simulink model "OpenLoop_TF_Asynch_Driver"  (R2021b)
settings: Solver=ode23s  StartTime=0.0  StopTime=10.0  MaxStep=10e-4  RelTol=1e-3  EnableMultiTasking=on
libraries: spsUniversalBridgeLib x2, spsVoltageMeasurementLib x2, spsAsynchronousMachineSIUnitsLib x1, spsCurrentMeasurementLib x1, spsPWMGenerator2LevelLib x1, spsRMSLib x1, simulink x1, spsSeriesRLCBranchLib x1, spsThreePhaseProgrammableVoltageSourceLib x1, spspowerguiLib x1
settings Model: Creator=Mostafa  LastModifiedBy=Unicorn
settings SolverCC: AlgebraicLoopSolver=TrustRegion
settings DataIOCC: ReturnWorkspaceOutputs=off
settings OptimizationCC: LifeSpan=inf
settings DebuggingCC: SFUnexpectedBacktrackingDiag=warning  SFNoUnconditionalDefaultTransitionDiag=warning  SFMachineParentedDataDiag=warning  ArithmeticOperatorsInVariantConditions=warning
settings SFSimCC: SimUseLocalCustomCode=off  CustomCodeUndefinedFunction=UseInterfaceOnly
settings RTWCC: RTWUseLocalCustomCode=off
settings CodeAppCC: StateflowObjectComments=on
settings GRTTargetCC: TargetLangStandard=C89/C90 (ANSI)
settings ConfigComp: CovMetricSettings=dw  CovSaveCumulativeToWorkspaceVar=on  CovSaveSingleToWorkspaceVar=on  CovExternalEMLEnable=off
settings SimscapeCC: SimscapeNormalizeSystem=off

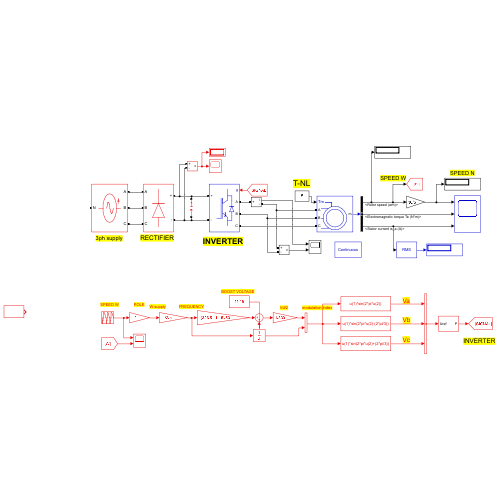
[thumbnail: Simulink's stored preview of the top-level diagram]
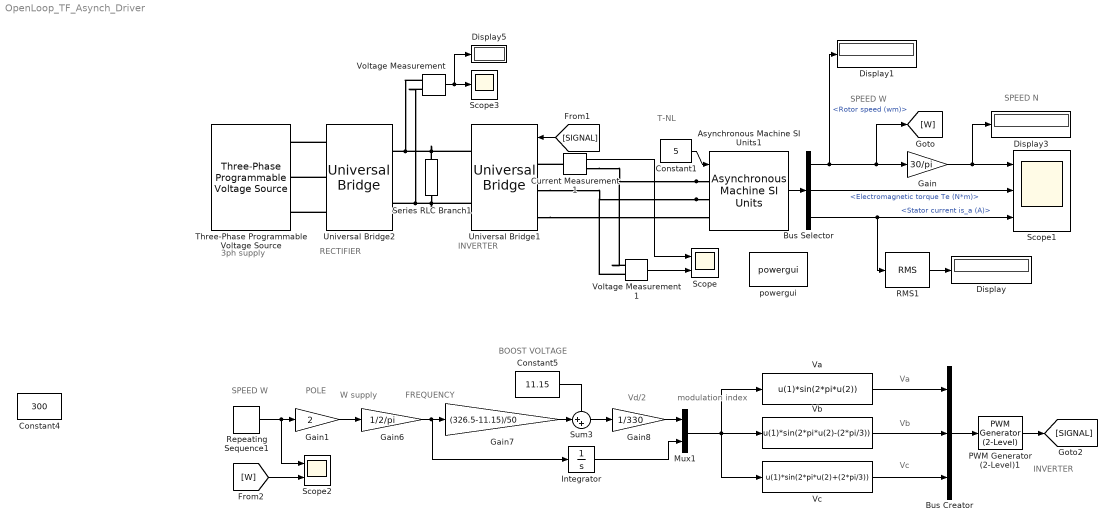
== system OpenLoop_TF_Asynch_Driver ==
  note: INVERTER
  note: Va
  note: RECTIFIER
  note: 3ph supply
  note: INVERTER
  note: T-NL
  note: SPEED W
  note: SPEED N
  note: POLE
  note: W supply
  note: BOOST VOLTAGE
  note: FREQUENCY
  note: SPEED W
  note: Vd/2
  note: modulation index
  note: Vb
  note: Vc
  Asynchronous Machine SI Units1 : spsAsynchronousMachineSIUnitsLib/Asynchronous Machine SI Units  RotorType=Squirrel-cage  PresetModel="15:  5.4 HP (4KW)   400 V  50Hz 1430 RPM"  MechanicalLoad=Torque Tm  ShowDetailedParameters=on  ReferenceFrame=Rotor  Units=SI  MeasurementBus=off  NominalParameters=[4000 400 50]  VoltageRatio=1  Stator=[1.405 0.005839]  Rotor=[1.395 0.005839]  Cage1=[0.4155 0.002066]  Cage2=[0.4168 0.0003495]  Lm=0.1722  Mechanical=[0.0131 0.002985 2]  PolePairs=2  InitialConditions=[1 0 0 0 0 0 0 0]  SimulateSaturation=off  Saturation=[14.03593122, 27.81365428, 53.79336849, 72.68890987, 97.98006896, 148.6815601, 215.7428561, 302.9841135, 428.7778367 ; 230, 322, 414, 460, 506, 552, 598, 644, 690]  LoadFlowParameters=1492000  TsPowergui=0  TsBlock=-1  IterativeModel=Trapezoidal non iterative  IterativeDiscreteModel=Trapezoidal non iterative  Pmec=1.492e+006
  Bus Creator : BusCreator  Inputs=3
  Bus Selector : BusSelector  OutputSignals=Mechanical.Rotor speed (wm),Mechanical.Electromagnetic torque Te (N*m),Stator measurements.Stator current is_a (A)
  Constant1 : Constant  Value=5
  Constant4 : Constant  Value=300
  Constant5 : Constant  Value=11.15
  Current Measurement1 : spsCurrentMeasurementLib/Current Measurement  PhasorSimulation=off  OutputType=Complex  PSBequivalent=0
  Display{,1,3,5} (4 alike) : Display
  Gain : Gain  Gain=30/pi
  Gain1 : Gain  Gain=2
  Gain6 : Gain  Gain=1/2/pi
  Gain7 : Gain  Gain=(326.5-11.15)/50
  Gain8 : Gain  Gain=1/330
  Integrator : Integrator
  Mux1 : Mux  Inputs=2
  PWM Generator (2-Level)1 : spsPWMGenerator2LevelLib/PWM Generator (2-Level)  ModulatorType=Three-phase bridge (6 pulses)  ModulatorMode=Unsynchronized  Fc=27*60  Pc=90  nF=27  MinMax="[ -1  1 ]"  SamplingTechnique=Natural  ModulatingSignals=off  m=0.8  Freq=60  Phase=0  Ts=0  ShowCarrierOutport=off
  RMS1 : spsRMSLib/RMS  TrueRMS=on  Freq=50  RMSInit=0  Ts=0
  Repeating Sequence1 : simulink/Sources/Repeating Sequence  rep_seq_t=[0 1 1.1 2 2.1 3 3.1 4 4.1 5 5.1 8 8.1 10]  rep_seq_y=[200 200 100 100 150 150 200 200 300 300 300 250 250 200]
  Scope : Scope  NumInputPorts=2
  Scope1 : Scope  NumInputPorts=3
  Scope2 : Scope  NumInputPorts=2
  Scope3 : Scope
  Series RLC Branch1 : spsSeriesRLCBranchLib/Series RLC Branch  LConnTagsString=__new0  RConnTagsString=__new0  BranchType=C  Resistance=1  Inductance=1e-3  SetiL0=off  InitialCurrent=0  Capacitance=50e-3  Setx0=off  InitialVoltage=0  Measurements=None
  Sum3 : Sum  Inputs=|++
  Three-Phase Programmable Voltage Source : spsThreePhaseProgrammableVoltageSourceLib/Three-Phase Programmable Voltage Source  PositiveSequence=[466.7 0 50]  VariationEntity=None  VariationType=Table of time-amplitude pairs  VariationTypeAlt=Step  VariationStep=0.5  VariationRate=10  VariationMagnitude=0.3  VariationFrequency=2  VariationTiming=[1 2]  VariationPhaseA=off  Amplitudes=[1 0.8 1.2 1.0]  TimeValues=[0 0.1 0.15 0.2]  HarmonicGeneration=off  HarmonicA=[3 0.2 -25 0]  HarmonicB=[2 0.15 35 2]  Timing="[0.05  3]"  BusType=swing  Pref=0  Qref=0  Qmin=-inf  Qmax=inf
  Universal Bridge1 : spsUniversalBridgeLib/Universal Bridge  Arms=3  SnubberResistance=1e5  SnubberCapacitance=inf  Device=IGBT / Diodes  Ron=1e-3  Lon=0  ForwardVoltages="[  0  0  ]"  ForwardVoltage=0  GTOparameters=[ 10e-6 , 20e-6 ]  IGBTparameters=[ 1e-6 , 2e-6 ]  Measurements=None  Measurements_2=None  converterType=Rectifier
  Universal Bridge2 : spsUniversalBridgeLib/Universal Bridge  Arms=3  SnubberResistance=1e5  SnubberCapacitance=inf  Device=Diodes  Ron=1e-3  Lon=0  ForwardVoltages="[  0  0  ]"  ForwardVoltage=0  GTOparameters=[ 10e-6 , 20e-6 ]  IGBTparameters=[ 1e-6 , 2e-6 ]  Measurements=None  Measurements_2=None  converterType=Rectifier
  Va : Fcn  Expr=u(1)*sin(2*pi*u(2))
  Vb : Fcn  Expr=u(1)*sin(2*pi*u(2)-(2*pi/3))
  Vc : Fcn  Expr=u(1)*sin(2*pi*u(2)+(2*pi/3))
  Voltage Measurement : spsVoltageMeasurementLib/Voltage Measurement  PhasorSimulation=off  OutputType=Complex  PSBequivalent=0
  Voltage Measurement1 : spsVoltageMeasurementLib/Voltage Measurement  PhasorSimulation=off  OutputType=Complex  PSBequivalent=0
  powergui : spspowerguiLib/powergui  Priority=1  SimulationMode=Continuous  SampleTime=10e-6  frequency=60  Iterations=50  frequencyindice=50  Pbase=100e6  ErrMax=1e-4  UnitsV=kV  UnitsW=MW  buscounter=0  FunctionMessages=off  echomessages=off  EnableUseOfTLC=off  CurrentSourceSwitches=on  DisableSnubberDevices=off  DisableRonSwitches=off  DisableVfSwitches=off  DisplayEquations=off  AutomaticDiscreteSolvers=off  SolverType=Tustin/Backward Euler (TBE)  Interpol=off  ExternalGateDelay=off  methode=off  Ts=10  x0status=blocks  SPID=off  SwTol=0  HookPort=off  NonlinearTolerance=1e-4  nMaxIteration=100  ContinueOnMaxIteration=off  RestoreLinks=warning  ResistiveCurrentMeasurement=off  Frange=[0:2:500]  Ylog=off  Xlog=on  ShowGrid=off  save=off  variable=ZData  structure=0  ZoomFFT=off  StartTime=0.0  cycles=1  DisplayStyle=1  fundamental=60  FreqAxis=off  MaxFrequency=1000  frequencyindicesteady=1  RmsSteady=1  display=off
  wires:
  Asynchronous Machine SI Units1/1 -> Bus Selector/1
  Bus Selector/1 -> Display1/1, [W], Gain/1  "<Rotor speed (wm)>"
  Bus Selector/2 -> Scope1/2  "<Electromagnetic torque Te (N*m)>"
  Bus Selector/3 -> RMS1/1, Scope1/3  "<Stator current is_a (A)>"
  RMS1/1 -> Display/1
  Voltage Measurement1/1 -> Scope/2
  Current Measurement1/1 -> Scope/1
  [SIGNAL] -> Universal Bridge1/1
  Gain/1 -> Display3/1, Scope1/1
  Constant1/1 -> Asynchronous Machine SI Units1/1
  Voltage Measurement/1 -> Display5/1, Scope3/1
  Repeating Sequence1/1 -> Scope2/1, Gain1/1
  Gain1/1 -> Gain6/1
  Gain6/1 -> Integrator/1, Gain7/1
  Gain7/1 -> Sum3/1
  Constant5/1 -> Sum3/2
  Sum3/1 -> Gain8/1
  Va/1 -> Bus Creator/1
  Vb/1 -> Bus Creator/2
  Vc/1 -> Bus Creator/3
  Bus Creator/1 -> PWM Generator (2-Level)1/1
  PWM Generator (2-Level)1/1 -> [SIGNAL]
  Gain8/1 -> Mux1/1
  Mux1/1 -> Vc/1, Va/1, Vb/1
  Integrator/1 -> Mux1/2
  [W] -> Scope2/2
  connections:
  Asynchronous Machine SI Units1/LConn1 -- Current Measurement1/RConn1 -- Voltage Measurement1/LConn1
  Asynchronous Machine SI Units1/LConn2 -- Universal Bridge1/LConn2 -- Voltage Measurement1/LConn2
  Series RLC Branch1/LConn1 -- Voltage Measurement/LConn1 -- Universal Bridge2/RConn1 -- Universal Bridge1/RConn1
  Series RLC Branch1/RConn1 -- Voltage Measurement/LConn2 -- Universal Bridge2/RConn2 -- Universal Bridge1/RConn2
  Universal Bridge1/LConn3 -- Asynchronous Machine SI Units1/LConn3
  Universal Bridge2/LConn1 -- Three-Phase Programmable Voltage Source/RConn1
  Current Measurement1/LConn1 -- Universal Bridge1/LConn1
  Universal Bridge2/LConn3 -- Three-Phase Programmable Voltage Source/RConn3
  Universal Bridge2/LConn2 -- Three-Phase Programmable Voltage Source/RConn2
